simulink model "automata_learning"  (R2022a)
settings: Solver=FixedStepAuto  StartTime=0.0  StopTime=10.0  FixedStep=0.05  RelTol=1e-3
settings Model: Creator=diego  LastModifiedBy=diego

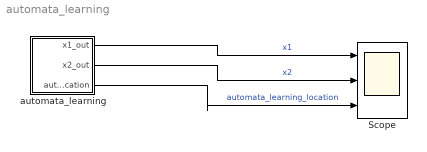
== system automata_learning ==
  Scope : Scope  NumInputPorts=3
  automata_learning : Stateflow chart  TreatAsAtomicUnit=on
  wires:
  automata_learning/1(x1_out) -> Scope/1  "x1"
  automata_learning/2(x2_out) -> Scope/2  "x2"
  automata_learning/3(automata_learning_location) -> Scope/3  "automata_learning_location"

== stateflow chart automata_learning/automata_learning ==
  settings: updateMethod=CONTINUOUS
  state loc1
    du:
    x1_dot = 0.3267960846424103 * (exp(1.0048383474349976 * x1 + 0.19207751750946045 * x2 + 0.14201068878173828) - 1.0) / (exp(1.0048383474349976 * x1 + 0.19207751750946045 * x2 + 0.14201068878173828) + 1.0) - 0.26445508003234863 * (exp(0.25733521580696106 * x1 + 0.6826767325401306 * x2 + 0.016339562833309174) - 1.0) / (exp(0.25733521580696106 * x1 + 0.6826767325401306 * x2 + 0.016339562833309174) + 1.0) + 0.42201241850852966 * (exp(0.3862309157848358 * x1 - 0.693699836730957 * x2 + 0.26673072576522827) - 1.0) / (exp(0.3862309157848358 * x1 - 0.693699836730957 * x2 + 0.26673072576522827) + 1.0) + 0.3632749021053314 * (exp(0.9873818159103394 * x1 + 0.6307393312454224 * x2 + 0.12534266710281372) - 1.0) / (exp(0.9873818159103394 * x1 + 0.6307393312454224 * x2 + 0.12534266710281372) + 1.0) + 0.10125888139009476 * (exp(0.20049560070037842 * x1 - 0.160559743642807 * x2 + 0.1824951469898224) - 1.0) / (exp(0.20049560070037842 * x1 - 0.160559743642807 * x2 + 0.1824951469898224) + 1.0) + 0.40173691511154175 * (exp(0.12253177165985107 * x1 + 0.5087800025939941 * x2 + 0.1722065806388855) - 1.0) / (exp(0.12253177165985107 * x1 + 0.5087800025939941 * x2 + 0.1722065806388855) + 1.0) + 0.3918328583240509 * (exp(0.77249675989151 * x1 + 0.23811350762844086 * x2 + 0.25376445055007935) - 1.0) / (exp(0.77249675989151 * x1 + 0.23811350762844086 * x2 + 0.25376445055007935) + 1.0) + 0.5315578579902649 * (exp(0.7527535557746887 * x2 - 0.71623295545578 * x1 + 0.1934361755847931) - 1.0) / (exp(0.7527535557746887 * x2 - 0.71623295545578 * x1 + 0.1934361755847931) + 1.0) + 0.21696101129055023 * (exp(1.145237922668457 * x1 - 0.48395270109176636 * x2 + 0.17693766951560974) - 1.0) / (exp(1.145237922668457 * x1 - 0.48395270109176636 * x2 + 0.17693766951560974) + 1.0) + 0.4498450458049774 * (exp(0.005149938631802797 * x2 - 0.7853907942771912 * x1 + 0.20130854845046997) - 1.0) / (exp(0.005149938631802797 * x2 - 0.7853907942771912 * x1 + 0.20130854845046997) + 1.0) + 0.3854547441005707 * (exp(0.0945829525589943 * x2 - 0.06022552028298378 * x1 + 0.13296866416931152) - 1.0) / (exp(0.0945829525589943 * x2 - 0.06022552028298378 * x1 + 0.13296866416931152) + 1.0) - 0.3562648594379425 * (exp(0.0715617835521698 * x1 + 0.23621444404125214 * x2 - 0.19701531529426575) - 1.0) / (exp(0.0715617835521698 * x1 + 0.23621444404125214 * x2 - 0.19701531529426575) + 1.0) + 0.01290080975741148 * (exp(0.16716276109218597 * x1 + 0.8158755898475647 * x2 - 0.05134623870253563) - 1.0) / (exp(0.16716276109218597 * x1 + 0.8158755898475647 * x2 - 0.05134623870253563) + 1.0) - 0.3389087915420532 * (exp(0.17453202605247498 * x1 + 0.3652767837047577 * x2 - 0.2213810831308365) - 1.0) / (exp(0.17453202605247498 * x1 + 0.3652767837047577 * x2 - 0.2213810831308365) + 1.0) + 0.4367385506629944 * (exp(0.3806522786617279 * x2 - 0.09918756037950516 * x1 + 0.1911337971687317) - 1.0) / (exp(0.3806522786617279 * x2 - 0.09918756037950516 * x1 + 0.1911337971687317) + 1.0) - 0.36950942873954773 * (exp(0.42811957001686096 * x1 + 0.3712623417377472 * x2 - 0.09048526734113693) - 1.0) / (exp(0.42811957001686096 * x1 + 0.3712623417377472 * x2 - 0.09048526734113693) + 1.0) + 0.2180066704750061 * (exp(0.5884444117546082 * x1 + 0.8796142935752869 * x2 + 0.1144915223121643) - 1.0) / (exp(0.5884444117546082 * x1 + 0.8796142935752869 * x2 + 0.1144915223121643) + 1.0) - 0.2895767092704773 * (exp(0.6668423414230347 * x1 + 0.8922714591026306 * x2 - 0.11080985516309738) - 1.0) / (exp(0.6668423414230347 * x1 + 0.8922714591026306 * x2 - 0.11080985516309738) + 1.0) - 0.07781984657049179 * (exp(0.8882426619529724 * x1 - 0.46987950801849365 * x2 + 0.16808292269706726) - 1.0) / (exp(0.8882426619529724 * x1 - 0.46987950801849365 * x2 + 0.16808292269706726) + 1.0) + 0.4442409873008728 * (exp(0.9243723750114441 * x1 + 1.2910957336425781 * x2 + 0.23949529230594635) - 1.0) / (exp(0.9243723750114441 * x1 + 1.2910957336425781 * x2 + 0.23949529230594635) + 1.0) + 0.03949417173862457;
    x2_dot = 0.5663174986839294 * (exp(0.25733521580696106 * x1 + 0.6826767325401306 * x2 + 0.016339562833309174) - 1.0) / (exp(0.25733521580696106 * x1 + 0.6826767325401306 * x2 + 0.016339562833309174) + 1.0) + 0.3859030604362488 * (exp(1.0048383474349976 * x1 + 0.19207751750946045 * x2 + 0.14201068878173828) - 1.0) / (exp(1.0048383474349976 * x1 + 0.19207751750946045 * x2 + 0.14201068878173828) + 1.0) - 0.3649897873401642 * (exp(0.3862309157848358 * x1 - 0.693699836730957 * x2 + 0.26673072576522827) - 1.0) / (exp(0.3862309157848358 * x1 - 0.693699836730957 * x2 + 0.26673072576522827) + 1.0) + 0.45027482509613037 * (exp(0.9873818159103394 * x1 + 0.6307393312454224 * x2 + 0.12534266710281372) - 1.0) / (exp(0.9873818159103394 * x1 + 0.6307393312454224 * x2 + 0.12534266710281372) + 1.0) - 0.00898544117808342 * (exp(0.20049560070037842 * x1 - 0.160559743642807 * x2 + 0.1824951469898224) - 1.0) / (exp(0.20049560070037842 * x1 - 0.160559743642807 * x2 + 0.1824951469898224) + 1.0) + 0.364576518535614 * (exp(0.12253177165985107 * x1 + 0.5087800025939941 * x2 + 0.1722065806388855) - 1.0) / (exp(0.12253177165985107 * x1 + 0.5087800025939941 * x2 + 0.1722065806388855) + 1.0) - 0.28657159209251404 * (exp(0.77249675989151 * x1 + 0.23811350762844086 * x2 + 0.25376445055007935) - 1.0) / (exp(0.77249675989151 * x1 + 0.23811350762844086 * x2 + 0.25376445055007935) + 1.0) + 0.3877284526824951 * (exp(0.7527535557746887 * x2 - 0.71623295545578 * x1 + 0.1934361755847931) - 1.0) / (exp(0.7527535557746887 * x2 - 0.71623295545578 * x1 + 0.1934361755847931) + 1.0) + 0.3060077726840973 * (exp(1.145237922668457 * x1 - 0.48395270109176636 * x2 + 0.17693766951560974) - 1.0) / (exp(1.145237922668457 * x1 - 0.48395270109176636 * x2 + 0.17693766951560974) + 1.0) - 0.5428471565246582 * (exp(0.005149938631802797 * x2 - 0.7853907942771912 * x1 + 0.20130854845046997) - 1.0) / (exp(0.005149938631802797 * x2 - 0.7853907942771912 * x1 + 0.20130854845046997) + 1.0) - 0.22001713514328003 * (exp(0.0945829525589943 * x2 - 0.06022552028298378 * x1 + 0.13296866416931152) - 1.0) / (exp(0.0945829525589943 * x2 - 0.06022552028298378 * x1 + 0.13296866416931152) + 1.0) - 0.16401030123233795 * (exp(0.0715617835521698 * x1 + 0.23621444404125214 * x2 - 0.19701531529426575) - 1.0) / (exp(0.0715617835521698 * x1 + 0.23621444404125214 * x2 - 0.19701531529426575) + 1.0) - 0.07008145749568939 * (exp(0.16716276109218597 * x1 + 0.8158755898475647 * x2 - 0.05134623870253563) - 1.0) / (exp(0.16716276109218597 * x1 + 0.8158755898475647 * x2 - 0.05134623870253563) + 1.0) + 0.014245678670704365 * (exp(0.17453202605247498 * x1 + 0.3652767837047577 * x2 - 0.2213810831308365) - 1.0) / (exp(0.17453202605247498 * x1 + 0.3652767837047577 * x2 - 0.2213810831308365) + 1.0) + 0.2984023094177246 * (exp(0.3806522786617279 * x2 - 0.09918756037950516 * x1 + 0.1911337971687317) - 1.0) / (exp(0.3806522786617279 * x2 - 0.09918756037950516 * x1 + 0.1911337971687317) + 1.0) + 0.4591461420059204 * (exp(0.42811957001686096 * x1 + 0.3712623417377472 * x2 - 0.09048526734113693) - 1.0) / (exp(0.42811957001686096 * x1 + 0.3712623417377472 * x2 - 0.09048526734113693) + 1.0) + 0.38253578543663025 * (exp(0.5884444117546082 * x1 + 0.8796142935752869 * x2 + 0.1144915223121643) - 1.0) / (exp(0.5884444117546082 * x1 + 0.8796142935752869 * x2 + 0.1144915223121643) + 1.0) - 0.3770252764225006 * (exp(0.6668423414230347 * x1 + 0.8922714591026306 * x2 - 0.11080985516309738) - 1.0) / (exp(0.6668423414230347 * x1 + 0.8922714591026306 * x2 - 0.11080985516309738) + 1.0) + 0.29143598675727844 * (exp(0.8882426619529724 * x1 - 0.46987950801849365 * x2 + 0.16808292269706726) - 1.0) / (exp(0.8882426619529724 * x1 - 0.46987950801849365 * x2 + 0.16808292269706726) + 1.0) - 0.2532555162906647 * (exp(0.9243723750114441 * x1 + 1.2910957336425781 * x2 + 0.23949529230594635) - 1.0) / (exp(0.9243723750114441 * x1 + 1.2910957336425781 * x2 + 0.23949529230594635) + 1.0) + 0.08314455300569534;
    x1_out=x1;
    x2_out=x2;
    automata_learning_location =1;
  state loc2
    du:
    x1_dot = 0.35343942046165466 * (exp(0.7641435861587524 * x1 - 0.45938730239868164 * x2 + 0.014588812366127968) - 1.0) / (exp(0.7641435861587524 * x1 - 0.45938730239868164 * x2 + 0.014588812366127968) + 1.0) + 0.1568225473165512 * (exp(0.17216528952121735 * x1 + 1.046384334564209 * x2 + 0.0010911826975643635) - 1.0) / (exp(0.17216528952121735 * x1 + 1.046384334564209 * x2 + 0.0010911826975643635) + 1.0) + 0.5362024903297424 * (exp(0.604775071144104 * x1 + 0.5488911867141724 * x2 + 0.07835572957992554) - 1.0) / (exp(0.604775071144104 * x1 + 0.5488911867141724 * x2 + 0.07835572957992554) + 1.0) + 0.1035316213965416 * (exp(0.19428350031375885 * x1 + 1.0496068000793457 * x2 + 0.03221691772341728) - 1.0) / (exp(0.19428350031375885 * x1 + 1.0496068000793457 * x2 + 0.03221691772341728) + 1.0) + 0.4003770649433136 * (exp(0.5251650214195251 * x1 + 0.0374409444630146 * x2 + 0.17754621803760529) - 1.0) / (exp(0.5251650214195251 * x1 + 0.0374409444630146 * x2 + 0.17754621803760529) + 1.0) - 0.5087916254997253 * (exp(0.6394046545028687 * x1 - 0.6333951354026794 * x2 + 0.07158142328262329) - 1.0) / (exp(0.6394046545028687 * x1 - 0.6333951354026794 * x2 + 0.07158142328262329) + 1.0) + 0.11881831288337708 * (exp(0.7476024627685547 * x1 - 0.5308956503868103 * x2 + 0.04502331465482712) - 1.0) / (exp(0.7476024627685547 * x1 - 0.5308956503868103 * x2 + 0.04502331465482712) + 1.0) - 0.2664828598499298 * (exp(0.8175243735313416 * x2 - 0.14570258557796478 * x1 + 0.0789196565747261) - 1.0) / (exp(0.8175243735313416 * x2 - 0.14570258557796478 * x1 + 0.0789196565747261) + 1.0) - 0.3760240375995636 * (exp(0.5433180332183838 * x1 + 0.061846088618040085 * x2 + 0.07081878185272217) - 1.0) / (exp(0.5433180332183838 * x1 + 0.061846088618040085 * x2 + 0.07081878185272217) + 1.0) - 0.4801105260848999 * (exp(0.6028870344161987 * x2 - 0.7738447189331055 * x1 + 0.09245716035366058) - 1.0) / (exp(0.6028870344161987 * x2 - 0.7738447189331055 * x1 + 0.09245716035366058) + 1.0) - 0.5020380616188049 * (exp(0.615638792514801 * x1 - 0.7856979370117188 * x2 + 0.18128538131713867) - 1.0) / (exp(0.615638792514801 * x1 - 0.7856979370117188 * x2 + 0.18128538131713867) + 1.0) - 0.31106022000312805 * (exp(0.08418424427509308 * x1 + 0.283954918384552 * x2 - 0.0308680459856987) - 1.0) / (exp(0.08418424427509308 * x1 + 0.283954918384552 * x2 - 0.0308680459856987) + 1.0) + 0.16113443672657013 * (exp(0.23439587652683258 * x1 + 0.389376699924469 * x2 + 0.06722152233123779) - 1.0) / (exp(0.23439587652683258 * x1 + 0.389376699924469 * x2 + 0.06722152233123779) + 1.0) - 0.12505723536014557 * (exp(0.8433523774147034 * x1 + 0.8931418657302856 * x2 - 0.06894798576831818) - 1.0) / (exp(0.8433523774147034 * x1 + 0.8931418657302856 * x2 - 0.06894798576831818) + 1.0) - 0.3894966244697571 * (exp(0.1163388341665268 * x1 + 1.0107378959655762 * x2 + 0.05383792519569397) - 1.0) / (exp(0.1163388341665268 * x1 + 1.0107378959655762 * x2 + 0.05383792519569397) + 1.0) - 0.42704156041145325 * (exp(0.6177901029586792 * x2 - 0.4676801562309265 * x1 + 0.01174979843199253) - 1.0) / (exp(0.6177901029586792 * x2 - 0.4676801562309265 * x1 + 0.01174979843199253) + 1.0) - 0.3586192727088928 * (exp(0.23055383563041687 * x1 - 0.3186957836151123 * x2 + 0.09966936707496643) - 1.0) / (exp(0.23055383563041687 * x1 - 0.3186957836151123 * x2 + 0.09966936707496643) + 1.0) - 0.22417937219142914 * (exp(0.3105676770210266 * x2 - 0.4884205162525177 * x1 + 0.09676644206047058) - 1.0) / (exp(0.3105676770210266 * x2 - 0.4884205162525177 * x1 + 0.09676644206047058) + 1.0) + 0.031713396310806274 * (exp(0.8288009762763977 * x1 - 0.9553812742233276 * x2 + 0.03843358904123306) - 1.0) / (exp(0.8288009762763977 * x1 - 0.9553812742233276 * x2 + 0.03843358904123306) + 1.0) - 0.3144373297691345 * (exp(0.6887566447257996 * x1 + 0.4987463057041168 * x2 - 0.10281724482774734) - 1.0) / (exp(0.6887566447257996 * x1 + 0.4987463057041168 * x2 - 0.10281724482774734) + 1.0) + 0.01631726697087288;
    x2_dot = 0.3543780744075775 * (exp(0.7641435861587524 * x1 - 0.45938730239868164 * x2 + 0.014588812366127968) - 1.0) / (exp(0.7641435861587524 * x1 - 0.45938730239868164 * x2 + 0.014588812366127968) + 1.0) + 0.35056835412979126 * (exp(0.17216528952121735 * x1 + 1.046384334564209 * x2 + 0.0010911826975643635) - 1.0) / (exp(0.17216528952121735 * x1 + 1.046384334564209 * x2 + 0.0010911826975643635) + 1.0) + 0.11538253724575043 * (exp(0.604775071144104 * x1 + 0.5488911867141724 * x2 + 0.07835572957992554) - 1.0) / (exp(0.604775071144104 * x1 + 0.5488911867141724 * x2 + 0.07835572957992554) + 1.0) + 0.5423222184181213 * (exp(0.19428350031375885 * x1 + 1.0496068000793457 * x2 + 0.03221691772341728) - 1.0) / (exp(0.19428350031375885 * x1 + 1.0496068000793457 * x2 + 0.03221691772341728) + 1.0) + 0.24572955071926117 * (exp(0.5251650214195251 * x1 + 0.0374409444630146 * x2 + 0.17754621803760529) - 1.0) / (exp(0.5251650214195251 * x1 + 0.0374409444630146 * x2 + 0.17754621803760529) + 1.0) - 0.5155855417251587 * (exp(0.6394046545028687 * x1 - 0.6333951354026794 * x2 + 0.07158142328262329) - 1.0) / (exp(0.6394046545028687 * x1 - 0.6333951354026794 * x2 + 0.07158142328262329) + 1.0) + 0.3996223211288452 * (exp(0.7476024627685547 * x1 - 0.5308956503868103 * x2 + 0.04502331465482712) - 1.0) / (exp(0.7476024627685547 * x1 - 0.5308956503868103 * x2 + 0.04502331465482712) + 1.0) + 0.0992613136768341 * (exp(0.8175243735313416 * x2 - 0.14570258557796478 * x1 + 0.0789196565747261) - 1.0) / (exp(0.8175243735313416 * x2 - 0.14570258557796478 * x1 + 0.0789196565747261) + 1.0) + 0.24699389934539795 * (exp(0.5433180332183838 * x1 + 0.061846088618040085 * x2 + 0.07081878185272217) - 1.0) / (exp(0.5433180332183838 * x1 + 0.061846088618040085 * x2 + 0.07081878185272217) + 1.0) + 0.19099585711956024 * (exp(0.6028870344161987 * x2 - 0.7738447189331055 * x1 + 0.09245716035366058) - 1.0) / (exp(0.6028870344161987 * x2 - 0.7738447189331055 * x1 + 0.09245716035366058) + 1.0) - 0.22115595638751984 * (exp(0.615638792514801 * x1 - 0.7856979370117188 * x2 + 0.18128538131713867) - 1.0) / (exp(0.615638792514801 * x1 - 0.7856979370117188 * x2 + 0.18128538131713867) + 1.0) + 0.03549620136618614 * (exp(0.08418424427509308 * x1 + 0.283954918384552 * x2 - 0.0308680459856987) - 1.0) / (exp(0.08418424427509308 * x1 + 0.283954918384552 * x2 - 0.0308680459856987) + 1.0) + 0.076938696205616 * (exp(0.23439587652683258 * x1 + 0.389376699924469 * x2 + 0.06722152233123779) - 1.0) / (exp(0.23439587652683258 * x1 + 0.389376699924469 * x2 + 0.06722152233123779) + 1.0) - 0.24228310585021973 * (exp(0.8433523774147034 * x1 + 0.8931418657302856 * x2 - 0.06894798576831818) - 1.0) / (exp(0.8433523774147034 * x1 + 0.8931418657302856 * x2 - 0.06894798576831818) + 1.0) - 0.17632551491260529 * (exp(0.1163388341665268 * x1 + 1.0107378959655762 * x2 + 0.05383792519569397) - 1.0) / (exp(0.1163388341665268 * x1 + 1.0107378959655762 * x2 + 0.05383792519569397) + 1.0) - 0.34705162048339844 * (exp(0.6177901029586792 * x2 - 0.4676801562309265 * x1 + 0.01174979843199253) - 1.0) / (exp(0.6177901029586792 * x2 - 0.4676801562309265 * x1 + 0.01174979843199253) + 1.0) + 0.3387020528316498 * (exp(0.23055383563041687 * x1 - 0.3186957836151123 * x2 + 0.09966936707496643) - 1.0) / (exp(0.23055383563041687 * x1 - 0.3186957836151123 * x2 + 0.09966936707496643) + 1.0) + 0.40590399503707886 * (exp(0.3105676770210266 * x2 - 0.4884205162525177 * x1 + 0.09676644206047058) - 1.0) / (exp(0.3105676770210266 * x2 - 0.4884205162525177 * x1 + 0.09676644206047058) + 1.0) + 0.22574880719184875 * (exp(0.8288009762763977 * x1 - 0.9553812742233276 * x2 + 0.03843358904123306) - 1.0) / (exp(0.8288009762763977 * x1 - 0.9553812742233276 * x2 + 0.03843358904123306) + 1.0) + 0.014472335577011108 * (exp(0.6887566447257996 * x1 + 0.4987463057041168 * x2 - 0.10281724482774734) - 1.0) / (exp(0.6887566447257996 * x1 + 0.4987463057041168 * x2 - 0.10281724482774734) + 1.0) + 0.08348819613456726;
    x1_out=x1;
    x2_out=x2;
    automata_learning_location =2;
  loc1 -> loc2 : [0.0000005511 * x2 - 0.2482 * x1 + 1.0 < 0.0]
  (default) -> loc1 : {x1 = 0.0;
      | x2 = 0.0;}
  loc2 -> loc1 : [43.09132960916031 * x1 + 0.021145646542095164 * x2 + 1.0 < 0.0 && -75.02048562094569 * x1 - 0.1991395009226835 * x2 + 1.0 > 0.0]
  data: x1_out output; x1 local; x2_out output; x2 local; automata_learning_location output
  data x1 settings: updateMethod=SF_CONTINUOUS_TIME_DATA
  data x2 settings: updateMethod=SF_CONTINUOUS_TIME_DATA
